simulink model "sampleModel7424_pp_1_1"  (R2018a)
settings: Solver=VariableStepAuto  StartTime=0.0  StopTime=10.0  RelTol=1e-3
undefined symbols (not defined in the file): DiscIntNeverNeededParam
libraries: simulink x211
(part 5 of 7)

== system sampleModel7424_pp_1_1/cfblk134/cfblk19 ==
  cfblk1 : Inport
  cfblk11 : Inport  Port=2
  cfblk12 : Inport  Port=3
  Action Port : ActionPort  ActionType=else
  cfblk10 : simulink/Continuous/PID Controller  Controller=PID  TimeDomain=Discrete-time  SampleTime=-1  IntegratorMethod=Forward Euler  FilterMethod=Forward Euler  Form=Parallel  UseFilter=on  ControllerParametersSource=internal  P=1  I=1  D=0  N=100  InitialConditionSource=internal  InitialConditionForIntegrator=0  InitialConditionForFilter=0  ExternalReset=none  LimitOutput=off  UpperSaturationLimit=inf  LowerSaturationLimit=-inf  LinearizeAsGain=off  AntiWindupMode=none  Kb=1  TrackingMode=off  Kt=1  PParamMin=[]  PParamMax=[]  IParamMin=[]  IParamMax=[]  DParamMin=[]  DParamMax=[]  NParamMin=[]  NParamMax=[]  KbParamMin=[]  KbParamMax=[]  KtParamMin=[]  KtParamMax=[]  POutMin=[]  POutMax=[]  IOutMin=[]  IOutMax=[]  DOutMin=[]  DOutMax=[]  NOutMin=[]  NOutMax=[]  KbOutMin=[]  KbOutMax=[]  KtOutMin=[]  KtOutMax=[]  IntegratorOutMin=[]  IntegratorOutMax=[]  FilterOutMin=[]  FilterOutMax=[]  SumOutMin=[]  SumOutMax=[]  SumI1OutMin=[]  SumI1OutMax=[]  SumI2OutMin=[]  SumI2OutMax=[]  SumI3OutMin=[]  SumI3OutMax=[]  SumDOutMin=[]  SumDOutMax=[]  SaturationOutMin=[]  SaturationOutMax=[]  IntegratorContinuousStateAttributes=''  IntegratorStateMustResolveToSignalObject=off  IntegratorRTWStateStorageClass=Auto  FilterContinuousStateAttributes=''  FilterStateMustResolveToSignalObject=off  FilterRTWStateStorageClass=Auto  DifferentiatorICPrevScaledInput=0  DifferentiatorOutMin=[]  DifferentiatorOutMax=[]  FilterDiffOutCoefMin=[]  FilterDiffOutCoefMax=[]  SumDenOutMin=[]  SumDenOutMax=[]  SumNumOutMin=[]  SumNumOutMax=[]  ReciprocalOutMin=[]  ReciprocalOutMax=[]  DivideOutMin=[]  DivideOutMax=[]  TunerSelectOption=Transfer Function Based (PID Tuner App)
  cfblk15 : Delay
  cfblk3 : simulink/Continuous/PID Controller (2DOF)  Controller=PID  TimeDomain=Discrete-time  SampleTime=-1  IntegratorMethod=Forward Euler  FilterMethod=Forward Euler  Form=Parallel  UseFilter=on  ControllerParametersSource=internal  P=1  I=1  D=0  N=100  b=1  c=1  InitialConditionSource=internal  InitialConditionForIntegrator=0  InitialConditionForFilter=0  ExternalReset=none  LimitOutput=off  UpperSaturationLimit=inf  LowerSaturationLimit=-inf  LinearizeAsGain=off  AntiWindupMode=none  Kb=1  TrackingMode=off  Kt=1  PParamMin=[]  PParamMax=[]  IParamMin=[]  IParamMax=[]  DParamMin=[]  DParamMax=[]  NParamMin=[]  NParamMax=[]  bParamMin=[]  bParamMax=[]  cParamMin=[]  cParamMax=[]  KbParamMin=[]  KbParamMax=[]  KtParamMin=[]  KtParamMax=[]  POutMin=[]  POutMax=[]  IOutMin=[]  IOutMax=[]  DOutMin=[]  DOutMax=[]  NOutMin=[]  NOutMax=[]  bOutMin=[]  bOutMax=[]  cOutMin=[]  cOutMax=[]  KbOutMin=[]  KbOutMax=[]  KtOutMin=[]  KtOutMax=[]  IntegratorOutMin=[]  IntegratorOutMax=[]  FilterOutMin=[]  FilterOutMax=[]  SumOutMin=[]  SumOutMax=[]  Sum1OutMin=[]  Sum1OutMax=[]  Sum2OutMin=[]  Sum2OutMax=[]  Sum3OutMin=[]  Sum3OutMax=[]  SumI1OutMin=[]  SumI1OutMax=[]  SumI2OutMin=[]  SumI2OutMax=[]  SumI3OutMin=[]  SumI3OutMax=[]  SumDOutMin=[]  SumDOutMax=[]  SaturationOutMin=[]  SaturationOutMax=[]  IntegratorContinuousStateAttributes=''  IntegratorStateMustResolveToSignalObject=off  IntegratorRTWStateStorageClass=Auto  FilterContinuousStateAttributes=''  FilterStateMustResolveToSignalObject=off  FilterRTWStateStorageClass=Auto  DifferentiatorICPrevScaledInput=0  DifferentiatorOutMin=[]  DifferentiatorOutMax=[]  FilterDiffOutCoefMin=[]  FilterDiffOutCoefMax=[]  SumDenOutMin=[]  SumDenOutMax=[]  SumNumOutMin=[]  SumNumOutMax=[]  ReciprocalOutMin=[]  ReciprocalOutMax=[]  DivideOutMin=[]  DivideOutMax=[]  TunerSelectOption=Transfer Function Based (PID Tuner App)
  cfblk4 : simulink/Continuous/PID Controller  Controller=PID  TimeDomain=Discrete-time  SampleTime=-1  IntegratorMethod=Forward Euler  FilterMethod=Forward Euler  Form=Parallel  UseFilter=on  ControllerParametersSource=internal  P=1  I=1  D=0  N=100  InitialConditionSource=internal  InitialConditionForIntegrator=0  InitialConditionForFilter=0  ExternalReset=none  LimitOutput=off  UpperSaturationLimit=inf  LowerSaturationLimit=-inf  LinearizeAsGain=off  AntiWindupMode=none  Kb=1  TrackingMode=off  Kt=1  PParamMin=[]  PParamMax=[]  IParamMin=[]  IParamMax=[]  DParamMin=[]  DParamMax=[]  NParamMin=[]  NParamMax=[]  KbParamMin=[]  KbParamMax=[]  KtParamMin=[]  KtParamMax=[]  POutMin=[]  POutMax=[]  IOutMin=[]  IOutMax=[]  DOutMin=[]  DOutMax=[]  NOutMin=[]  NOutMax=[]  KbOutMin=[]  KbOutMax=[]  KtOutMin=[]  KtOutMax=[]  IntegratorOutMin=[]  IntegratorOutMax=[]  FilterOutMin=[]  FilterOutMax=[]  SumOutMin=[]  SumOutMax=[]  SumI1OutMin=[]  SumI1OutMax=[]  SumI2OutMin=[]  SumI2OutMax=[]  SumI3OutMin=[]  SumI3OutMax=[]  SumDOutMin=[]  SumDOutMax=[]  SaturationOutMin=[]  SaturationOutMax=[]  IntegratorContinuousStateAttributes=''  IntegratorStateMustResolveToSignalObject=off  IntegratorRTWStateStorageClass=Auto  FilterContinuousStateAttributes=''  FilterStateMustResolveToSignalObject=off  FilterRTWStateStorageClass=Auto  DifferentiatorICPrevScaledInput=0  DifferentiatorOutMin=[]  DifferentiatorOutMax=[]  FilterDiffOutCoefMin=[]  FilterDiffOutCoefMax=[]  SumDenOutMin=[]  SumDenOutMax=[]  SumNumOutMin=[]  SumNumOutMax=[]  ReciprocalOutMin=[]  ReciprocalOutMax=[]  DivideOutMin=[]  DivideOutMax=[]  TunerSelectOption=Transfer Function Based (PID Tuner App)
  cfblk5 : DiscreteFir
  cfblk6 : DiscreteFilter
  cfblk7 : DiscreteFir
  cfblk8 : simulink/Discrete/Difference  ICPrevInput=0.0  OutMin=[]  OutMax=[]  OutDataTypeStr=double  OutputDataTypeScalingMode=double  OutDataType=fixdt(1, 16)  OutScaling=2^-10  DoSatur=off
  cfblk9 : simulink/Discrete/Tapped Delay  vinit=0.0  samptime=-1  NumDelays=1  DelayOrder=Oldest  includeCurrent=off
  cyemi_{417..426} (10 alike) : DataTypeConversion  OutDataTypeStr=double
  emi_{68,76,148,276,282,298} (6 alike) : UnaryMinus
  emi_149 : MATLAB Function  TreatAsAtomicUnit=on
  emi_277 : MATLAB Function  TreatAsAtomicUnit=on
  emi_283 : MATLAB Function  TreatAsAtomicUnit=on
  emi_299 : MATLAB Function  TreatAsAtomicUnit=on
  emi_69 : MATLAB Function  TreatAsAtomicUnit=on
  emi_77 : MATLAB Function  TreatAsAtomicUnit=on
  cfblk2 : Outport
  cfblk13 : Outport  Port=2
  cfblk14 : Outport  Port=3
  wires:
  cfblk4/1 -> cfblk13/1, cfblk2/1
  cfblk12/1 -> cfblk14/1
  cyemi_417/1 -> cfblk10/1, emi_276/1, emi_277/1(o)
  cfblk8/1 -> cyemi_417/1
  cyemi_418/1 -> cfblk15/1
  cfblk9/1 -> cyemi_418/1
  cyemi_419/1 -> cfblk3/1
  cfblk10/1 -> cyemi_419/1
  cyemi_420/1 -> cfblk3/2
  cfblk7/1 -> cyemi_420/1
  cyemi_421/1 -> cfblk4/1
  cfblk3/1 -> cyemi_421/1
  cyemi_422/1 -> cfblk5/1, emi_148/1, emi_149/1(o)
  cfblk15/1 -> cyemi_422/1
  cyemi_423/1 -> cfblk6/1, emi_282/1, emi_283/1(o)
  cfblk11/1 -> cyemi_423/1
  cyemi_424/1 -> cfblk7/1, emi_68/1, emi_69/1(o), emi_298/1, emi_299/1(o)
  cfblk1/1 -> cyemi_424/1
  cyemi_425/1 -> cfblk8/1
  cfblk6/1 -> cyemi_425/1
  cyemi_426/1 -> cfblk9/1, emi_76/1, emi_77/1(o)
  cfblk5/1 -> cyemi_426/1
  emi_68/1 -> emi_69/2(e)
  emi_76/1 -> emi_77/2(e)
  emi_148/1 -> emi_149/2(e)
  emi_276/1 -> emi_277/2(e)
  emi_282/1 -> emi_283/2(e)
  emi_298/1 -> emi_299/2(e)

== system sampleModel7424_pp_1_1/cfblk142/cfblk16 ==
  cfblk1 : Inport
  cfblk11 : Inport  Port=2
  Action Port : ActionPort  ActionType=then
  cfblk10 : simulink/Discrete/Transfer Fcn First Order  PoleZ=0.95  ICPrevOutput=0.0  DoSatur=off
      settings: SourceProductName=Simulink
  cfblk12 : Delay
  cfblk3 : simulink/Continuous/PID Controller (2DOF)  Controller=PID  TimeDomain=Discrete-time  SampleTime=-1  IntegratorMethod=Forward Euler  FilterMethod=Forward Euler  Form=Parallel  UseFilter=on  ControllerParametersSource=internal  P=1  I=1  D=0  N=100  b=1  c=1  InitialConditionSource=internal  InitialConditionForIntegrator=0  InitialConditionForFilter=0  ExternalReset=none  LimitOutput=off  UpperSaturationLimit=inf  LowerSaturationLimit=-inf  LinearizeAsGain=off  AntiWindupMode=none  Kb=1  TrackingMode=off  Kt=1  PParamMin=[]  PParamMax=[]  IParamMin=[]  IParamMax=[]  DParamMin=[]  DParamMax=[]  NParamMin=[]  NParamMax=[]  bParamMin=[]  bParamMax=[]  cParamMin=[]  cParamMax=[]  KbParamMin=[]  KbParamMax=[]  KtParamMin=[]  KtParamMax=[]  POutMin=[]  POutMax=[]  IOutMin=[]  IOutMax=[]  DOutMin=[]  DOutMax=[]  NOutMin=[]  NOutMax=[]  bOutMin=[]  bOutMax=[]  cOutMin=[]  cOutMax=[]  KbOutMin=[]  KbOutMax=[]  KtOutMin=[]  KtOutMax=[]  IntegratorOutMin=[]  IntegratorOutMax=[]  FilterOutMin=[]  FilterOutMax=[]  SumOutMin=[]  SumOutMax=[]  Sum1OutMin=[]  Sum1OutMax=[]  Sum2OutMin=[]  Sum2OutMax=[]  Sum3OutMin=[]  Sum3OutMax=[]  SumI1OutMin=[]  SumI1OutMax=[]  SumI2OutMin=[]  SumI2OutMax=[]  SumI3OutMin=[]  SumI3OutMax=[]  SumDOutMin=[]  SumDOutMax=[]  SaturationOutMin=[]  SaturationOutMax=[]  IntegratorContinuousStateAttributes=''  IntegratorStateMustResolveToSignalObject=off  IntegratorRTWStateStorageClass=Auto  FilterContinuousStateAttributes=''  FilterStateMustResolveToSignalObject=off  FilterRTWStateStorageClass=Auto  DifferentiatorICPrevScaledInput=0  DifferentiatorOutMin=[]  DifferentiatorOutMax=[]  FilterDiffOutCoefMin=[]  FilterDiffOutCoefMax=[]  SumDenOutMin=[]  SumDenOutMax=[]  SumNumOutMin=[]  SumNumOutMax=[]  ReciprocalOutMin=[]  ReciprocalOutMax=[]  DivideOutMin=[]  DivideOutMax=[]  TunerSelectOption=Transfer Function Based (PID Tuner App)
  cfblk4 : simulink/Continuous/PID Controller (2DOF)  Controller=PID  TimeDomain=Discrete-time  SampleTime=-1  IntegratorMethod=Forward Euler  FilterMethod=Forward Euler  Form=Parallel  UseFilter=on  ControllerParametersSource=internal  P=1  I=1  D=0  N=100  b=1  c=1  InitialConditionSource=internal  InitialConditionForIntegrator=0  InitialConditionForFilter=0  ExternalReset=none  LimitOutput=off  UpperSaturationLimit=inf  LowerSaturationLimit=-inf  LinearizeAsGain=off  AntiWindupMode=none  Kb=1  TrackingMode=off  Kt=1  PParamMin=[]  PParamMax=[]  IParamMin=[]  IParamMax=[]  DParamMin=[]  DParamMax=[]  NParamMin=[]  NParamMax=[]  bParamMin=[]  bParamMax=[]  cParamMin=[]  cParamMax=[]  KbParamMin=[]  KbParamMax=[]  KtParamMin=[]  KtParamMax=[]  POutMin=[]  POutMax=[]  IOutMin=[]  IOutMax=[]  DOutMin=[]  DOutMax=[]  NOutMin=[]  NOutMax=[]  bOutMin=[]  bOutMax=[]  cOutMin=[]  cOutMax=[]  KbOutMin=[]  KbOutMax=[]  KtOutMin=[]  KtOutMax=[]  IntegratorOutMin=[]  IntegratorOutMax=[]  FilterOutMin=[]  FilterOutMax=[]  SumOutMin=[]  SumOutMax=[]  Sum1OutMin=[]  Sum1OutMax=[]  Sum2OutMin=[]  Sum2OutMax=[]  Sum3OutMin=[]  Sum3OutMax=[]  SumI1OutMin=[]  SumI1OutMax=[]  SumI2OutMin=[]  SumI2OutMax=[]  SumI3OutMin=[]  SumI3OutMax=[]  SumDOutMin=[]  SumDOutMax=[]  SaturationOutMin=[]  SaturationOutMax=[]  IntegratorContinuousStateAttributes=''  IntegratorStateMustResolveToSignalObject=off  IntegratorRTWStateStorageClass=Auto  FilterContinuousStateAttributes=''  FilterStateMustResolveToSignalObject=off  FilterRTWStateStorageClass=Auto  DifferentiatorICPrevScaledInput=0  DifferentiatorOutMin=[]  DifferentiatorOutMax=[]  FilterDiffOutCoefMin=[]  FilterDiffOutCoefMax=[]  SumDenOutMin=[]  SumDenOutMax=[]  SumNumOutMin=[]  SumNumOutMax=[]  ReciprocalOutMin=[]  ReciprocalOutMax=[]  DivideOutMin=[]  DivideOutMax=[]  TunerSelectOption=Transfer Function Based (PID Tuner App)
  cfblk5 : Delay  DelayLengthSource=Input port
      settings: InputPortMap=u0,p1
  cfblk6 : simulink/Discrete/Tapped Delay  vinit=0.0  samptime=-1  NumDelays=1  DelayOrder=Oldest  includeCurrent=off
  cfblk7 : DiscreteFir
  cfblk8 : simulink/Discrete/Tapped Delay  vinit=0.0  samptime=-1  NumDelays=1  DelayOrder=Oldest  includeCurrent=off
  cfblk9 : simulink/Continuous/PID Controller (2DOF)  Controller=PID  TimeDomain=Discrete-time  SampleTime=-1  IntegratorMethod=Forward Euler  FilterMethod=Forward Euler  Form=Parallel  UseFilter=on  ControllerParametersSource=internal  P=1  I=1  D=0  N=100  b=1  c=1  InitialConditionSource=internal  InitialConditionForIntegrator=0  InitialConditionForFilter=0  ExternalReset=none  LimitOutput=off  UpperSaturationLimit=inf  LowerSaturationLimit=-inf  LinearizeAsGain=off  AntiWindupMode=none  Kb=1  TrackingMode=off  Kt=1  PParamMin=[]  PParamMax=[]  IParamMin=[]  IParamMax=[]  DParamMin=[]  DParamMax=[]  NParamMin=[]  NParamMax=[]  bParamMin=[]  bParamMax=[]  cParamMin=[]  cParamMax=[]  KbParamMin=[]  KbParamMax=[]  KtParamMin=[]  KtParamMax=[]  POutMin=[]  POutMax=[]  IOutMin=[]  IOutMax=[]  DOutMin=[]  DOutMax=[]  NOutMin=[]  NOutMax=[]  bOutMin=[]  bOutMax=[]  cOutMin=[]  cOutMax=[]  KbOutMin=[]  KbOutMax=[]  KtOutMin=[]  KtOutMax=[]  IntegratorOutMin=[]  IntegratorOutMax=[]  FilterOutMin=[]  FilterOutMax=[]  SumOutMin=[]  SumOutMax=[]  Sum1OutMin=[]  Sum1OutMax=[]  Sum2OutMin=[]  Sum2OutMax=[]  Sum3OutMin=[]  Sum3OutMax=[]  SumI1OutMin=[]  SumI1OutMax=[]  SumI2OutMin=[]  SumI2OutMax=[]  SumI3OutMin=[]  SumI3OutMax=[]  SumDOutMin=[]  SumDOutMax=[]  SaturationOutMin=[]  SaturationOutMax=[]  IntegratorContinuousStateAttributes=''  IntegratorStateMustResolveToSignalObject=off  IntegratorRTWStateStorageClass=Auto  FilterContinuousStateAttributes=''  FilterStateMustResolveToSignalObject=off  FilterRTWStateStorageClass=Auto  DifferentiatorICPrevScaledInput=0  DifferentiatorOutMin=[]  DifferentiatorOutMax=[]  FilterDiffOutCoefMin=[]  FilterDiffOutCoefMax=[]  SumDenOutMin=[]  SumDenOutMax=[]  SumNumOutMin=[]  SumNumOutMax=[]  ReciprocalOutMin=[]  ReciprocalOutMax=[]  DivideOutMin=[]  DivideOutMax=[]  TunerSelectOption=Transfer Function Based (PID Tuner App)
  cyemi_{528..540} (13 alike) : DataTypeConversion  OutDataTypeStr=double
  cfblk2 : Outport
  wires:
  cfblk9/1 -> cyemi_532/1, cyemi_538/1
  cfblk7/1 -> cyemi_528/1, cyemi_529/1
  cfblk5/1 -> cfblk2/1
  cfblk11/1 -> cyemi_533/1, cyemi_540/1
  cyemi_528/1 -> cfblk10/1
  cyemi_529/1 -> cfblk12/1
  cyemi_530/1 -> cfblk3/1
  cfblk1/1 -> cyemi_530/1
  cyemi_531/1 -> cfblk3/2
  cfblk12/1 -> cyemi_531/1
  cyemi_532/1 -> cfblk4/1
  cyemi_533/1 -> cfblk4/2
  cyemi_534/1 -> cfblk5/1
  cfblk8/1 -> cyemi_534/1
  cyemi_535/1 -> cfblk5/2
  cfblk4/1 -> cyemi_535/1
  cyemi_536/1 -> cfblk6/1
  cfblk3/1 -> cyemi_536/1
  cyemi_537/1 -> cfblk7/1
  cfblk6/1 -> cyemi_537/1
  cyemi_538/1 -> cfblk8/1
  cyemi_539/1 -> cfblk9/1
  cfblk10/1 -> cyemi_539/1
  cyemi_540/1 -> cfblk9/2

== system sampleModel7424_pp_1_1/cfblk142/cfblk17 ==
  cfblk1 : Inport
  Action Port : ActionPort  ActionType=else
  cfblk3 : simulink/Discrete/Difference  ICPrevInput=0.0  OutMin=[]  OutMax=[]  OutDataTypeStr=double  OutputDataTypeScalingMode=double  OutDataType=fixdt(1, 16)  OutScaling=2^-10  DoSatur=off
  cfblk4 : simulink/Discrete/Transfer Fcn Real Zero  ZeroZ=0.75  ICPrevInput=0.0  DoSatur=off
      settings: SourceProductName=Simulink  SourceProductBaseCode=SL
  cfblk5 : simulink/Discrete/Tapped Delay  vinit=0.0  samptime=-1  NumDelays=1  DelayOrder=Oldest  includeCurrent=off
  cfblk6 : simulink/Discrete/Transfer Fcn First Order  PoleZ=0.95  ICPrevOutput=0.0  DoSatur=off
      settings: SourceProductName=Simulink
  cfblk8 : Delay
  cyemi_{542..546} (5 alike) : DataTypeConversion  OutDataTypeStr=double
  emi_0 : UnaryMinus
  emi_1 : MATLAB Function  TreatAsAtomicUnit=on
  emi_74 : UnaryMinus
  emi_75 : MATLAB Function  TreatAsAtomicUnit=on
  emi_80 : UnaryMinus
  emi_81 : MATLAB Function  TreatAsAtomicUnit=on
  cfblk2 : Outport
  cfblk7 : Outport  Port=2
  wires:
  cfblk5/1 -> cfblk2/1
  cfblk1/1 -> cfblk7/1
  cfblk4/1 -> cyemi_544/1, cyemi_545/1
  cyemi_542/1 -> cfblk3/1, emi_80/1, emi_81/1(o)
  cfblk8/1 -> cyemi_542/1
  cyemi_543/1 -> cfblk4/1, emi_0/1, emi_1/1(o)
  cfblk3/1 -> cyemi_543/1
  cyemi_544/1 -> cfblk5/1
  cyemi_545/1 -> cfblk6/1
  cyemi_546/1 -> cfblk8/1, emi_74/1, emi_75/1(o)
  cfblk6/1 -> cyemi_546/1
  emi_0/1 -> emi_1/2(e)
  emi_74/1 -> emi_75/2(e)
  emi_80/1 -> emi_81/2(e)

== system sampleModel7424_pp_1_1/cfblk142/cfblk18 ==
  cfblk1 : Inport
  Action Port : ActionPort  ActionType=then
  cfblk10 : Delay  DelayLengthSource=Input port
      settings: InputPortMap=u0,p1
  cfblk11 : DiscreteStateSpace  SampleTime=-1
  cfblk12 : DiscreteFilter
  cfblk13 : simulink/Continuous/PID Controller  Controller=PID  TimeDomain=Discrete-time  SampleTime=-1  IntegratorMethod=Forward Euler  FilterMethod=Forward Euler  Form=Parallel  UseFilter=on  ControllerParametersSource=internal  P=1  I=1  D=0  N=100  InitialConditionSource=internal  InitialConditionForIntegrator=0  InitialConditionForFilter=0  ExternalReset=none  LimitOutput=off  UpperSaturationLimit=inf  LowerSaturationLimit=-inf  LinearizeAsGain=off  AntiWindupMode=none  Kb=1  TrackingMode=off  Kt=1  PParamMin=[]  PParamMax=[]  IParamMin=[]  IParamMax=[]  DParamMin=[]  DParamMax=[]  NParamMin=[]  NParamMax=[]  KbParamMin=[]  KbParamMax=[]  KtParamMin=[]  KtParamMax=[]  POutMin=[]  POutMax=[]  IOutMin=[]  IOutMax=[]  DOutMin=[]  DOutMax=[]  NOutMin=[]  NOutMax=[]  KbOutMin=[]  KbOutMax=[]  KtOutMin=[]  KtOutMax=[]  IntegratorOutMin=[]  IntegratorOutMax=[]  FilterOutMin=[]  FilterOutMax=[]  SumOutMin=[]  SumOutMax=[]  SumI1OutMin=[]  SumI1OutMax=[]  SumI2OutMin=[]  SumI2OutMax=[]  SumI3OutMin=[]  SumI3OutMax=[]  SumDOutMin=[]  SumDOutMax=[]  SaturationOutMin=[]  SaturationOutMax=[]  IntegratorContinuousStateAttributes=''  IntegratorStateMustResolveToSignalObject=off  IntegratorRTWStateStorageClass=Auto  FilterContinuousStateAttributes=''  FilterStateMustResolveToSignalObject=off  FilterRTWStateStorageClass=Auto  DifferentiatorICPrevScaledInput=0  DifferentiatorOutMin=[]  DifferentiatorOutMax=[]  FilterDiffOutCoefMin=[]  FilterDiffOutCoefMax=[]  SumDenOutMin=[]  SumDenOutMax=[]  SumNumOutMin=[]  SumNumOutMax=[]  ReciprocalOutMin=[]  ReciprocalOutMax=[]  DivideOutMin=[]  DivideOutMax=[]  TunerSelectOption=Transfer Function Based (PID Tuner App)
  cfblk{5,16..18} (4 alike) : Delay
  cfblk3 : Delay  ShowEnablePort=on
      settings: InputPortMap=u0,e6
  cfblk4 : simulink/Continuous/PID Controller (2DOF)  Controller=PID  TimeDomain=Discrete-time  SampleTime=-1  IntegratorMethod=Forward Euler  FilterMethod=Forward Euler  Form=Parallel  UseFilter=on  ControllerParametersSource=internal  P=1  I=1  D=0  N=100  b=1  c=1  InitialConditionSource=internal  InitialConditionForIntegrator=0  InitialConditionForFilter=0  ExternalReset=none  LimitOutput=off  UpperSaturationLimit=inf  LowerSaturationLimit=-inf  LinearizeAsGain=off  AntiWindupMode=none  Kb=1  TrackingMode=off  Kt=1  PParamMin=[]  PParamMax=[]  IParamMin=[]  IParamMax=[]  DParamMin=[]  DParamMax=[]  NParamMin=[]  NParamMax=[]  bParamMin=[]  bParamMax=[]  cParamMin=[]  cParamMax=[]  KbParamMin=[]  KbParamMax=[]  KtParamMin=[]  KtParamMax=[]  POutMin=[]  POutMax=[]  IOutMin=[]  IOutMax=[]  DOutMin=[]  DOutMax=[]  NOutMin=[]  NOutMax=[]  bOutMin=[]  bOutMax=[]  cOutMin=[]  cOutMax=[]  KbOutMin=[]  KbOutMax=[]  KtOutMin=[]  KtOutMax=[]  IntegratorOutMin=[]  IntegratorOutMax=[]  FilterOutMin=[]  FilterOutMax=[]  SumOutMin=[]  SumOutMax=[]  Sum1OutMin=[]  Sum1OutMax=[]  Sum2OutMin=[]  Sum2OutMax=[]  Sum3OutMin=[]  Sum3OutMax=[]  SumI1OutMin=[]  SumI1OutMax=[]  SumI2OutMin=[]  SumI2OutMax=[]  SumI3OutMin=[]  SumI3OutMax=[]  SumDOutMin=[]  SumDOutMax=[]  SaturationOutMin=[]  SaturationOutMax=[]  IntegratorContinuousStateAttributes=''  IntegratorStateMustResolveToSignalObject=off  IntegratorRTWStateStorageClass=Auto  FilterContinuousStateAttributes=''  FilterStateMustResolveToSignalObject=off  FilterRTWStateStorageClass=Auto  DifferentiatorICPrevScaledInput=0  DifferentiatorOutMin=[]  DifferentiatorOutMax=[]  FilterDiffOutCoefMin=[]  FilterDiffOutCoefMax=[]  SumDenOutMin=[]  SumDenOutMax=[]  SumNumOutMin=[]  SumNumOutMax=[]  ReciprocalOutMin=[]  ReciprocalOutMax=[]  DivideOutMin=[]  DivideOutMax=[]  TunerSelectOption=Transfer Function Based (PID Tuner App)
  cfblk6 : DiscreteTransferFcn
  cfblk7 : DiscreteTransferFcn
  cfblk8 : DiscreteFilter
  cfblk9 : DiscreteFir
  cyemi_{548..564} (17 alike) : DataTypeConversion  OutDataTypeStr=double
  cfblk2 : Outport
  cfblk14 : Outport  Port=2
  cfblk15 : Outport  Port=3
  wires:
  cfblk6/1 -> cfblk2/1
  cfblk5/1 -> cfblk14/1
  cfblk4/1 -> cfblk15/1
  cfblk9/1 -> cyemi_554/1, cyemi_555/1, cyemi_562/1
  cfblk11/1 -> cyemi_551/1, cyemi_558/1, cyemi_561/1
  cfblk7/1 -> cyemi_552/1, cyemi_553/1
  cyemi_548/1 -> cfblk10/1
  cfblk12/1 -> cyemi_548/1
  cyemi_549/1 -> cfblk10/2
  cfblk17/1 -> cyemi_549/1
  cyemi_550/1 -> cfblk11/1
  cfblk3/1 -> cyemi_550/1
  cyemi_551/1 -> cfblk12/1
  cyemi_552/1 -> cfblk13/1
  cyemi_553/1 -> cfblk16/1
  cyemi_554/1 -> cfblk17/1
  cyemi_555/1 -> cfblk18/1
  cyemi_556/1 -> cfblk3/1
  cfblk16/1 -> cyemi_556/1
  cyemi_557/1 -> cfblk3/2
  cfblk18/1 -> cyemi_557/1
  cyemi_558/1 -> cfblk4/1
  cyemi_559/1 -> cfblk4/2
  cfblk8/1 -> cyemi_559/1
  cyemi_560/1 -> cfblk5/1
  cfblk1/1 -> cyemi_560/1
  cyemi_561/1 -> cfblk6/1
  cyemi_562/1 -> cfblk7/1
  cyemi_563/1 -> cfblk8/1
  cfblk13/1 -> cyemi_563/1
  cyemi_564/1 -> cfblk9/1
  cfblk10/1 -> cyemi_564/1

== system sampleModel7424_pp_1_1/cfblk142/cfblk19 ==
  cfblk1 : Inport
  cfblk11 : Inport  Port=2
  Action Port : ActionPort  ActionType=else
  cfblk10 : DiscreteStateSpace  SampleTime=-1
  cfblk14 : Delay
  cfblk3 : simulink/Discrete/Transfer Fcn Real Zero  ZeroZ=0.75  ICPrevInput=0.0  DoSatur=off
      settings: SourceProductName=Simulink  SourceProductBaseCode=SL
  cfblk4 : DiscreteFilter
  cfblk5 : Delay  DelayLengthSource=Input port
      settings: InputPortMap=u0,p1
  cfblk6 : simulink/Continuous/PID Controller  Controller=PID  TimeDomain=Discrete-time  SampleTime=-1  IntegratorMethod=Forward Euler  FilterMethod=Forward Euler  Form=Parallel  UseFilter=on  ControllerParametersSource=internal  P=1  I=1  D=0  N=100  InitialConditionSource=internal  InitialConditionForIntegrator=0  InitialConditionForFilter=0  ExternalReset=none  LimitOutput=off  UpperSaturationLimit=inf  LowerSaturationLimit=-inf  LinearizeAsGain=off  AntiWindupMode=none  Kb=1  TrackingMode=off  Kt=1  PParamMin=[]  PParamMax=[]  IParamMin=[]  IParamMax=[]  DParamMin=[]  DParamMax=[]  NParamMin=[]  NParamMax=[]  KbParamMin=[]  KbParamMax=[]  KtParamMin=[]  KtParamMax=[]  POutMin=[]  POutMax=[]  IOutMin=[]  IOutMax=[]  DOutMin=[]  DOutMax=[]  NOutMin=[]  NOutMax=[]  KbOutMin=[]  KbOutMax=[]  KtOutMin=[]  KtOutMax=[]  IntegratorOutMin=[]  IntegratorOutMax=[]  FilterOutMin=[]  FilterOutMax=[]  SumOutMin=[]  SumOutMax=[]  SumI1OutMin=[]  SumI1OutMax=[]  SumI2OutMin=[]  SumI2OutMax=[]  SumI3OutMin=[]  SumI3OutMax=[]  SumDOutMin=[]  SumDOutMax=[]  SaturationOutMin=[]  SaturationOutMax=[]  IntegratorContinuousStateAttributes=''  IntegratorStateMustResolveToSignalObject=off  IntegratorRTWStateStorageClass=Auto  FilterContinuousStateAttributes=''  FilterStateMustResolveToSignalObject=off  FilterRTWStateStorageClass=Auto  DifferentiatorICPrevScaledInput=0  DifferentiatorOutMin=[]  DifferentiatorOutMax=[]  FilterDiffOutCoefMin=[]  FilterDiffOutCoefMax=[]  SumDenOutMin=[]  SumDenOutMax=[]  SumNumOutMin=[]  SumNumOutMax=[]  ReciprocalOutMin=[]  ReciprocalOutMax=[]  DivideOutMin=[]  DivideOutMax=[]  TunerSelectOption=Transfer Function Based (PID Tuner App)
  cfblk7 : DiscreteZeroPole  Poles=[0 0.5]  Gain=1  SampleTime=-1
  cfblk8 : DiscreteFilter
  cfblk9 : simulink/Discrete/Tapped Delay  vinit=0.0  samptime=-1  NumDelays=1  DelayOrder=Oldest  includeCurrent=off
  cyemi_{567..576} (10 alike) : DataTypeConversion  OutDataTypeStr=double
  emi_{8,10,56,86,170,212} (6 alike) : UnaryMinus
  emi_11 : MATLAB Function  TreatAsAtomicUnit=on
  emi_171 : MATLAB Function  TreatAsAtomicUnit=on
  emi_213 : MATLAB Function  TreatAsAtomicUnit=on
  emi_57 : MATLAB Function  TreatAsAtomicUnit=on
  emi_87 : MATLAB Function  TreatAsAtomicUnit=on
  emi_9 : MATLAB Function  TreatAsAtomicUnit=on
  cfblk2 : Outport
  cfblk12 : Outport  Port=2
  cfblk13 : Outport  Port=3
  wires:
  cfblk4/1 -> cfblk2/1, cfblk13/1
  cfblk8/1 -> cfblk12/1, cyemi_572/1
  cyemi_567/1 -> cfblk10/1
  cfblk3/1 -> cyemi_567/1
  cyemi_568/1 -> cfblk14/1
  cfblk7/1 -> cyemi_568/1
  cyemi_569/1 -> cfblk3/1, emi_8/1, emi_9/1(o), emi_86/1, emi_87/1(o)
  cfblk9/1 -> cyemi_569/1
  cyemi_570/1 -> cfblk4/1
  cfblk11/1 -> cyemi_570/1
  cyemi_571/1 -> cfblk5/1, emi_10/1, emi_11/1(o), emi_170/1, emi_171/1(o), emi_212/1, emi_213/1(o)
  cfblk14/1 -> cyemi_571/1
  cyemi_572/1 -> cfblk5/2
  cyemi_573/1 -> cfblk6/1
  cfblk10/1 -> cyemi_573/1
  cyemi_574/1 -> cfblk7/1
  cfblk6/1 -> cyemi_574/1
  cyemi_575/1 -> cfblk8/1
  cfblk1/1 -> cyemi_575/1
  cyemi_576/1 -> cfblk9/1, emi_56/1, emi_57/1(o)
  cfblk5/1 -> cyemi_576/1
  emi_8/1 -> emi_9/2(e)
  emi_10/1 -> emi_11/2(e)
  emi_56/1 -> emi_57/2(e)
  emi_86/1 -> emi_87/2(e)
  emi_170/1 -> emi_171/2(e)
  emi_212/1 -> emi_213/2(e)

== system sampleModel7424_pp_1_1/cfblk145/cfblk17 ==
  cfblk1 : Inport
  cfblk14 : Inport  Port=2
  cfblk15 : Inport  Port=3
  cfblk16 : Inport  Port=4
  Action Port : ActionPort  ActionType=then
  cfblk10 : DiscreteTransferFcn
  cfblk{3,5,11,13} (4 alike) : Delay  DelayLengthSource=Input port
      settings: InputPortMap=u0,p1
  cfblk12 : simulink/Discrete/Transfer Fcn Lead or Lag  PoleZ=0.95  ZeroZ=0.75  ICPrevOutput=0.0  ICPrevInput=0.0  DoSatur=off
      settings: SourceProductName=Simulink  SourceProductBaseCode=SL
  cfblk18 : Delay
  cfblk19 : DataTypeConversion  OutDataTypeStr=double
  cfblk20 : DataTypeConversion  OutDataTypeStr=double
  cfblk21 : DataTypeConversion  OutDataTypeStr=uint32
  cfblk22 : DataTypeConversion  OutDataTypeStr=double
  cfblk4 : DiscreteIntegrator  SampleTime=-1  OutDataTypeStr=double  ICPrevOutput=DiscIntNeverNeededParam  ICPrevScaledInput=DiscIntNeverNeededParam
  cfblk6 : DiscreteTransferFcn
  cfblk7 : simulink/Continuous/PID Controller (2DOF)  Controller=PID  TimeDomain=Discrete-time  SampleTime=-1  IntegratorMethod=Forward Euler  FilterMethod=Forward Euler  Form=Parallel  UseFilter=on  ControllerParametersSource=internal  P=1  I=1  D=0  N=100  b=1  c=1  InitialConditionSource=internal  InitialConditionForIntegrator=0  InitialConditionForFilter=0  ExternalReset=none  LimitOutput=off  UpperSaturationLimit=inf  LowerSaturationLimit=-inf  LinearizeAsGain=off  AntiWindupMode=none  Kb=1  TrackingMode=off  Kt=1  PParamMin=[]  PParamMax=[]  IParamMin=[]  IParamMax=[]  DParamMin=[]  DParamMax=[]  NParamMin=[]  NParamMax=[]  bParamMin=[]  bParamMax=[]  cParamMin=[]  cParamMax=[]  KbParamMin=[]  KbParamMax=[]  KtParamMin=[]  KtParamMax=[]  POutMin=[]  POutMax=[]  IOutMin=[]  IOutMax=[]  DOutMin=[]  DOutMax=[]  NOutMin=[]  NOutMax=[]  bOutMin=[]  bOutMax=[]  cOutMin=[]  cOutMax=[]  KbOutMin=[]  KbOutMax=[]  KtOutMin=[]  KtOutMax=[]  IntegratorOutMin=[]  IntegratorOutMax=[]  FilterOutMin=[]  FilterOutMax=[]  SumOutMin=[]  SumOutMax=[]  Sum1OutMin=[]  Sum1OutMax=[]  Sum2OutMin=[]  Sum2OutMax=[]  Sum3OutMin=[]  Sum3OutMax=[]  SumI1OutMin=[]  SumI1OutMax=[]  SumI2OutMin=[]  SumI2OutMax=[]  SumI3OutMin=[]  SumI3OutMax=[]  SumDOutMin=[]  SumDOutMax=[]  SaturationOutMin=[]  SaturationOutMax=[]  IntegratorContinuousStateAttributes=''  IntegratorStateMustResolveToSignalObject=off  IntegratorRTWStateStorageClass=Auto  FilterContinuousStateAttributes=''  FilterStateMustResolveToSignalObject=off  FilterRTWStateStorageClass=Auto  DifferentiatorICPrevScaledInput=0  DifferentiatorOutMin=[]  DifferentiatorOutMax=[]  FilterDiffOutCoefMin=[]  FilterDiffOutCoefMax=[]  SumDenOutMin=[]  SumDenOutMax=[]  SumNumOutMin=[]  SumNumOutMax=[]  ReciprocalOutMin=[]  ReciprocalOutMax=[]  DivideOutMin=[]  DivideOutMax=[]  TunerSelectOption=Transfer Function Based (PID Tuner App)
  cfblk8 : DiscreteFir
  cfblk9 : simulink/Discrete/Transfer Fcn Real Zero  ZeroZ=0.75  ICPrevInput=0.0  DoSatur=off
      settings: SourceProductName=Simulink  SourceProductBaseCode=SL
  cyemi_{626..627,629..633,635..646} (19 alike) : DataTypeConversion  OutDataTypeStr=double
  cyemi_628 : DataTypeConversion  OutDataTypeStr=uint32
  cyemi_634 : DataTypeConversion  OutDataTypeStr=uint32
  cfblk2 : Outport
  cfblk17 : Outport  Port=2
  wires:
  cfblk3/1 -> cfblk2/1
  cfblk1/1 -> cyemi_638/1, cyemi_641/1
  cfblk11/1 -> cfblk17/1
  cfblk8/1 -> cyemi_632/1, cyemi_636/1
  cfblk21/1 -> cyemi_628/1, cyemi_634/1
  cyemi_626/1 -> cfblk10/1
  cfblk16/1 -> cyemi_626/1
  cyemi_627/1 -> cfblk11/1
  cfblk10/1 -> cyemi_627/1
  cyemi_628/1 -> cfblk11/2
  cyemi_629/1 -> cfblk12/1
  cfblk22/1 -> cyemi_629/1
  cyemi_630/1 -> cfblk13/1
  cfblk19/1 -> cyemi_630/1
  cyemi_631/1 -> cfblk13/2
  cfblk4/1 -> cyemi_631/1
  cyemi_632/1 -> cfblk18/1
  cyemi_633/1 -> cfblk19/1
  cfblk9/1 -> cyemi_633/1
  cyemi_634/1 -> cfblk20/1
  cyemi_635/1 -> cfblk21/1
  cfblk12/1 -> cyemi_635/1
  cyemi_636/1 -> cfblk22/1
  cyemi_637/1 -> cfblk3/1
  cfblk13/1 -> cyemi_637/1
  cyemi_638/1 -> cfblk3/2
  cyemi_639/1 -> cfblk4/1
  cfblk7/1 -> cyemi_639/1
  cyemi_640/1 -> cfblk5/1
  cfblk14/1 -> cyemi_640/1
  cyemi_641/1 -> cfblk5/2
  cyemi_642/1 -> cfblk6/1
  cfblk18/1 -> cyemi_642/1
  cyemi_643/1 -> cfblk7/1
  cfblk15/1 -> cyemi_643/1
  cyemi_644/1 -> cfblk7/2
  cfblk5/1 -> cyemi_644/1
  cyemi_645/1 -> cfblk8/1
  cfblk6/1 -> cyemi_645/1
  cyemi_646/1 -> cfblk9/1
  cfblk20/1 -> cyemi_646/1

== system sampleModel7424_pp_1_1/cfblk145/cfblk18 ==
  cfblk1 : Inport
  cfblk15 : Inport  Port=2
  Action Port : ActionPort  ActionType=else
  cfblk10 : DiscreteStateSpace  SampleTime=-1
  cfblk11 : DiscreteIntegrator  SampleTime=-1  OutDataTypeStr=double  ICPrevOutput=DiscIntNeverNeededParam  ICPrevScaledInput=DiscIntNeverNeededParam
  cfblk12 : Delay  DelayLengthSource=Input port
      settings: InputPortMap=u0,p1
  cfblk13 : simulink/Continuous/PID Controller  Controller=PID  TimeDomain=Discrete-time  SampleTime=-1  IntegratorMethod=Forward Euler  FilterMethod=Forward Euler  Form=Parallel  UseFilter=on  ControllerParametersSource=internal  P=1  I=1  D=0  N=100  InitialConditionSource=internal  InitialConditionForIntegrator=0  InitialConditionForFilter=0  ExternalReset=none  LimitOutput=off  UpperSaturationLimit=inf  LowerSaturationLimit=-inf  LinearizeAsGain=off  AntiWindupMode=none  Kb=1  TrackingMode=off  Kt=1  PParamMin=[]  PParamMax=[]  IParamMin=[]  IParamMax=[]  DParamMin=[]  DParamMax=[]  NParamMin=[]  NParamMax=[]  KbParamMin=[]  KbParamMax=[]  KtParamMin=[]  KtParamMax=[]  POutMin=[]  POutMax=[]  IOutMin=[]  IOutMax=[]  DOutMin=[]  DOutMax=[]  NOutMin=[]  NOutMax=[]  KbOutMin=[]  KbOutMax=[]  KtOutMin=[]  KtOutMax=[]  IntegratorOutMin=[]  IntegratorOutMax=[]  FilterOutMin=[]  FilterOutMax=[]  SumOutMin=[]  SumOutMax=[]  SumI1OutMin=[]  SumI1OutMax=[]  SumI2OutMin=[]  SumI2OutMax=[]  SumI3OutMin=[]  SumI3OutMax=[]  SumDOutMin=[]  SumDOutMax=[]  SaturationOutMin=[]  SaturationOutMax=[]  IntegratorContinuousStateAttributes=''  IntegratorStateMustResolveToSignalObject=off  IntegratorRTWStateStorageClass=Auto  FilterContinuousStateAttributes=''  FilterStateMustResolveToSignalObject=off  FilterRTWStateStorageClass=Auto  DifferentiatorICPrevScaledInput=0  DifferentiatorOutMin=[]  DifferentiatorOutMax=[]  FilterDiffOutCoefMin=[]  FilterDiffOutCoefMax=[]  SumDenOutMin=[]  SumDenOutMax=[]  SumNumOutMin=[]  SumNumOutMax=[]  ReciprocalOutMin=[]  ReciprocalOutMax=[]  DivideOutMin=[]  DivideOutMax=[]  TunerSelectOption=Transfer Function Based (PID Tuner App)
  cfblk14 : simulink/Discrete/Difference  ICPrevInput=0.0  OutMin=[]  OutMax=[]  OutDataTypeStr=double  OutputDataTypeScalingMode=double  OutDataType=fixdt(1, 16)  OutScaling=2^-10  DoSatur=off
  cfblk16 : Delay
  cfblk17 : Delay
  cfblk18 : Delay
  cfblk3 : DiscreteFilter
  cfblk4 : Delay  ShowEnablePort=on
      settings: InputPortMap=u0,e6
  cfblk5 : DiscreteTransferFcn
  cfblk6 : simulink/Discrete/Transfer Fcn Lead or Lag  PoleZ=0.95  ZeroZ=0.75  ICPrevOutput=0.0  ICPrevInput=0.0  DoSatur=off
      settings: SourceProductName=Simulink  SourceProductBaseCode=SL
  cfblk7 : simulink/Discrete/Transfer Fcn Real Zero  ZeroZ=0.75  ICPrevInput=0.0  DoSatur=off
      settings: SourceProductName=Simulink  SourceProductBaseCode=SL
  cfblk8 : Delay  DelayLengthSource=Input port
      settings: InputPortMap=u0,p1
  cfblk9 : DiscreteIntegrator  SampleTime=-1  OutDataTypeStr=double  ICPrevOutput=DiscIntNeverNeededParam  ICPrevScaledInput=DiscIntNeverNeededParam
  cyemi_{649..666} (18 alike) : DataTypeConversion  OutDataTypeStr=double
  cfblk2 : Outport
  wires:
  cfblk11/1 -> cyemi_657/1, cyemi_664/1, cyemi_665/1
  cfblk3/1 -> cfblk2/1
  cyemi_649/1 -> cfblk10/1
  cfblk12/1 -> cyemi_649/1
  cyemi_650/1 -> cfblk11/1
  cfblk7/1 -> cyemi_650/1
  cyemi_651/1 -> cfblk12/1
  cfblk13/1 -> cyemi_651/1
  cyemi_652/1 -> cfblk12/2
  cfblk4/1 -> cyemi_652/1
  cyemi_653/1 -> cfblk13/1
  cfblk8/1 -> cyemi_653/1
  cyemi_654/1 -> cfblk14/1
  cfblk15/1 -> cyemi_654/1
  cyemi_655/1 -> cfblk16/1
  cfblk10/1 -> cyemi_655/1
  cyemi_656/1 -> cfblk17/1
  cfblk9/1 -> cyemi_656/1
  cyemi_657/1 -> cfblk18/1
  cyemi_658/1 -> cfblk3/1
  cfblk14/1 -> cyemi_658/1
  cyemi_659/1 -> cfblk4/1
  cfblk5/1 -> cyemi_659/1
  cyemi_660/1 -> cfblk4/2
  cfblk16/1 -> cyemi_660/1
  cyemi_661/1 -> cfblk5/1
  cfblk1/1 -> cyemi_661/1
  cyemi_662/1 -> cfblk6/1
  cfblk17/1 -> cyemi_662/1
  cyemi_663/1 -> cfblk7/1
  cfblk18/1 -> cyemi_663/1
  cyemi_664/1 -> cfblk8/1
  cyemi_665/1 -> cfblk8/2
  cyemi_666/1 -> cfblk9/1
  cfblk6/1 -> cyemi_666/1

== system sampleModel7424_pp_1_1/cfblk145/cfblk19 ==
  cfblk1 : Inport
  cfblk11 : Inport  Port=2
  Action Port : ActionPort  ActionType=then
  cfblk10 : DiscreteIntegrator  SampleTime=-1  OutDataTypeStr=double  ICPrevOutput=DiscIntNeverNeededParam  ICPrevScaledInput=DiscIntNeverNeededParam
  cfblk3 : UnitDelay  SampleTime=-1
  cfblk4 : simulink/Discrete/Difference  ICPrevInput=0.0  OutMin=[]  OutMax=[]  OutDataTypeStr=double  OutputDataTypeScalingMode=double  OutDataType=fixdt(1, 16)  OutScaling=2^-10  DoSatur=off
  cfblk5 : simulink/Discrete/Tapped Delay  vinit=0.0  samptime=-1  NumDelays=1  DelayOrder=Oldest  includeCurrent=off
  cfblk6 : simulink/Discrete/Transfer Fcn Real Zero  ZeroZ=0.75  ICPrevInput=0.0  DoSatur=off
      settings: SourceProductName=Simulink  SourceProductBaseCode=SL
  cfblk7 : simulink/Discrete/Tapped Delay  vinit=0.0  samptime=-1  NumDelays=1  DelayOrder=Oldest  includeCurrent=off
  cfblk8 : DiscreteStateSpace  SampleTime=-1
  cfblk9 : simulink/Continuous/PID Controller  Controller=PID  TimeDomain=Discrete-time  SampleTime=-1  IntegratorMethod=Forward Euler  FilterMethod=Forward Euler  Form=Parallel  UseFilter=on  ControllerParametersSource=internal  P=1  I=1  D=0  N=100  InitialConditionSource=internal  InitialConditionForIntegrator=0  InitialConditionForFilter=0  ExternalReset=none  LimitOutput=off  UpperSaturationLimit=inf  LowerSaturationLimit=-inf  LinearizeAsGain=off  AntiWindupMode=none  Kb=1  TrackingMode=off  Kt=1  PParamMin=[]  PParamMax=[]  IParamMin=[]  IParamMax=[]  DParamMin=[]  DParamMax=[]  NParamMin=[]  NParamMax=[]  KbParamMin=[]  KbParamMax=[]  KtParamMin=[]  KtParamMax=[]  POutMin=[]  POutMax=[]  IOutMin=[]  IOutMax=[]  DOutMin=[]  DOutMax=[]  NOutMin=[]  NOutMax=[]  KbOutMin=[]  KbOutMax=[]  KtOutMin=[]  KtOutMax=[]  IntegratorOutMin=[]  IntegratorOutMax=[]  FilterOutMin=[]  FilterOutMax=[]  SumOutMin=[]  SumOutMax=[]  SumI1OutMin=[]  SumI1OutMax=[]  SumI2OutMin=[]  SumI2OutMax=[]  SumI3OutMin=[]  SumI3OutMax=[]  SumDOutMin=[]  SumDOutMax=[]  SaturationOutMin=[]  SaturationOutMax=[]  IntegratorContinuousStateAttributes=''  IntegratorStateMustResolveToSignalObject=off  IntegratorRTWStateStorageClass=Auto  FilterContinuousStateAttributes=''  FilterStateMustResolveToSignalObject=off  FilterRTWStateStorageClass=Auto  DifferentiatorICPrevScaledInput=0  DifferentiatorOutMin=[]  DifferentiatorOutMax=[]  FilterDiffOutCoefMin=[]  FilterDiffOutCoefMax=[]  SumDenOutMin=[]  SumDenOutMax=[]  SumNumOutMin=[]  SumNumOutMax=[]  ReciprocalOutMin=[]  ReciprocalOutMax=[]  DivideOutMin=[]  DivideOutMax=[]  TunerSelectOption=Transfer Function Based (PID Tuner App)
  cyemi_{669..676} (8 alike) : DataTypeConversion  OutDataTypeStr=double
  cfblk2 : Outport
  cfblk12 : Outport  Port=2
  wires:
  cfblk1/1 -> cfblk12/1
  cfblk9/1 -> cfblk2/1
  cyemi_669/1 -> cfblk10/1
  cfblk5/1 -> cyemi_669/1
  cyemi_670/1 -> cfblk3/1
  cfblk10/1 -> cyemi_670/1
  cyemi_671/1 -> cfblk4/1
  cfblk8/1 -> cyemi_671/1
  cyemi_672/1 -> cfblk5/1
  cfblk6/1 -> cyemi_672/1
  cyemi_673/1 -> cfblk6/1
  cfblk4/1 -> cyemi_673/1
  cyemi_674/1 -> cfblk7/1
  cfblk3/1 -> cyemi_674/1
  cyemi_675/1 -> cfblk8/1
  cfblk11/1 -> cyemi_675/1
  cyemi_676/1 -> cfblk9/1
  cfblk7/1 -> cyemi_676/1

== system sampleModel7424_pp_1_1/cfblk145/cfblk20 ==
  cfblk1 : Inport
  cfblk10 : Inport  Port=2
  cfblk11 : Inport  Port=3
  cfblk12 : Inport  Port=4
  cfblk13 : Inport  Port=5
  Action Port : ActionPort  ActionType=else
  cfblk3 : simulink/Discrete/Difference  ICPrevInput=0.0  OutMin=[]  OutMax=[]  OutDataTypeStr=double  OutputDataTypeScalingMode=double  OutDataType=fixdt(1, 16)  OutScaling=2^-10  DoSatur=off
  cfblk4 : DiscreteFir
  cfblk5 : Delay
  cfblk6 : Delay
  cfblk7 : Delay  DelayLengthSource=Input port
      settings: InputPortMap=u0,p1
  cfblk8 : Delay  ShowEnablePort=on
      settings: InputPortMap=u0,e6
  cfblk9 : simulink/Discrete/Transfer Fcn Lead or Lag  PoleZ=0.95  ZeroZ=0.75  ICPrevOutput=0.0  ICPrevInput=0.0  DoSatur=off
      settings: SourceProductName=Simulink  SourceProductBaseCode=SL
  cyemi_{682..690} (9 alike) : DataTypeConversion  OutDataTypeStr=double
  cfblk2 : Outport
  cfblk14 : Outport  Port=2
  cfblk15 : Outport  Port=3
  wires:
  cfblk1/1 -> cfblk15/1
  cfblk12/1 -> cfblk2/1
  cfblk3/1 -> cfblk14/1
  cyemi_682/1 -> cfblk3/1
  cfblk5/1 -> cyemi_682/1
  cyemi_683/1 -> cfblk4/1
  cfblk6/1 -> cyemi_683/1
  cyemi_684/1 -> cfblk5/1
  cfblk9/1 -> cyemi_684/1
  cyemi_685/1 -> cfblk6/1
  cfblk11/1 -> cyemi_685/1
  cyemi_686/1 -> cfblk7/1
  cfblk4/1 -> cyemi_686/1
  cyemi_687/1 -> cfblk7/2
  cfblk10/1 -> cyemi_687/1
  cyemi_688/1 -> cfblk8/1
  cfblk13/1 -> cyemi_688/1
  cyemi_689/1 -> cfblk8/2
  cfblk7/1 -> cyemi_689/1
  cyemi_690/1 -> cfblk9/1
  cfblk8/1 -> cyemi_690/1

== system sampleModel7424_pp_1_1/cfblk148/cfblk18 ==
  cfblk1 : Inport
  Action Port : ActionPort  ActionType=then
  cfblk11 : DataTypeConversion  OutDataTypeStr=double
  cfblk12 : DataTypeConversion  OutDataTypeStr=uint32
  cfblk13 : DataTypeConversion  OutDataTypeStr=uint32
  cfblk14 : DataTypeConversion  OutDataTypeStr=double
  cfblk3 : DiscreteFir
  cfblk4 : simulink/Continuous/PID Controller  Controller=PID  TimeDomain=Discrete-time  SampleTime=-1  IntegratorMethod=Forward Euler  FilterMethod=Forward Euler  Form=Parallel  UseFilter=on  ControllerParametersSource=internal  P=1  I=1  D=0  N=100  InitialConditionSource=internal  InitialConditionForIntegrator=0  InitialConditionForFilter=0  ExternalReset=none  LimitOutput=off  UpperSaturationLimit=inf  LowerSaturationLimit=-inf  LinearizeAsGain=off  AntiWindupMode=none  Kb=1  TrackingMode=off  Kt=1  PParamMin=[]  PParamMax=[]  IParamMin=[]  IParamMax=[]  DParamMin=[]  DParamMax=[]  NParamMin=[]  NParamMax=[]  KbParamMin=[]  KbParamMax=[]  KtParamMin=[]  KtParamMax=[]  POutMin=[]  POutMax=[]  IOutMin=[]  IOutMax=[]  DOutMin=[]  DOutMax=[]  NOutMin=[]  NOutMax=[]  KbOutMin=[]  KbOutMax=[]  KtOutMin=[]  KtOutMax=[]  IntegratorOutMin=[]  IntegratorOutMax=[]  FilterOutMin=[]  FilterOutMax=[]  SumOutMin=[]  SumOutMax=[]  SumI1OutMin=[]  SumI1OutMax=[]  SumI2OutMin=[]  SumI2OutMax=[]  SumI3OutMin=[]  SumI3OutMax=[]  SumDOutMin=[]  SumDOutMax=[]  SaturationOutMin=[]  SaturationOutMax=[]  IntegratorContinuousStateAttributes=''  IntegratorStateMustResolveToSignalObject=off  IntegratorRTWStateStorageClass=Auto  FilterContinuousStateAttributes=''  FilterStateMustResolveToSignalObject=off  FilterRTWStateStorageClass=Auto  DifferentiatorICPrevScaledInput=0  DifferentiatorOutMin=[]  DifferentiatorOutMax=[]  FilterDiffOutCoefMin=[]  FilterDiffOutCoefMax=[]  SumDenOutMin=[]  SumDenOutMax=[]  SumNumOutMin=[]  SumNumOutMax=[]  ReciprocalOutMin=[]  ReciprocalOutMax=[]  DivideOutMin=[]  DivideOutMax=[]  TunerSelectOption=Transfer Function Based (PID Tuner App)
  cfblk5 : DiscreteZeroPole  Poles=[0 0.5]  Gain=1  SampleTime=-1
  cfblk6 : DiscreteFir
  cfblk7 : DiscreteTransferFcn
  cfblk8 : DiscreteStateSpace  SampleTime=-1
  cyemi_743 : DataTypeConversion  OutDataTypeStr=uint32
  cyemi_{744..752} (9 alike) : DataTypeConversion  OutDataTypeStr=double
  cfblk2 : Outport
  cfblk9 : Outport  Port=2
  cfblk10 : Outport  Port=3
  wires:
  cfblk3/1 -> cyemi_746/1, cyemi_752/1
  cfblk5/1 -> cfblk9/1, cyemi_751/1
  cfblk12/1 -> cfblk2/1
  cfblk13/1 -> cfblk10/1
  cyemi_743/1 -> cfblk11/1
  cfblk1/1 -> cyemi_743/1
  cyemi_744/1 -> cfblk12/1
  cfblk8/1 -> cyemi_744/1
  cyemi_745/1 -> cfblk13/1
  cfblk4/1 -> cyemi_745/1
  cyemi_746/1 -> cfblk14/1
  cyemi_747/1 -> cfblk3/1
  cfblk6/1 -> cyemi_747/1
  cyemi_748/1 -> cfblk4/1
  cfblk14/1 -> cyemi_748/1
  cyemi_749/1 -> cfblk5/1
  cfblk11/1 -> cyemi_749/1
  cyemi_750/1 -> cfblk6/1
  cfblk7/1 -> cyemi_750/1
  cyemi_751/1 -> cfblk7/1
  cyemi_752/1 -> cfblk8/1

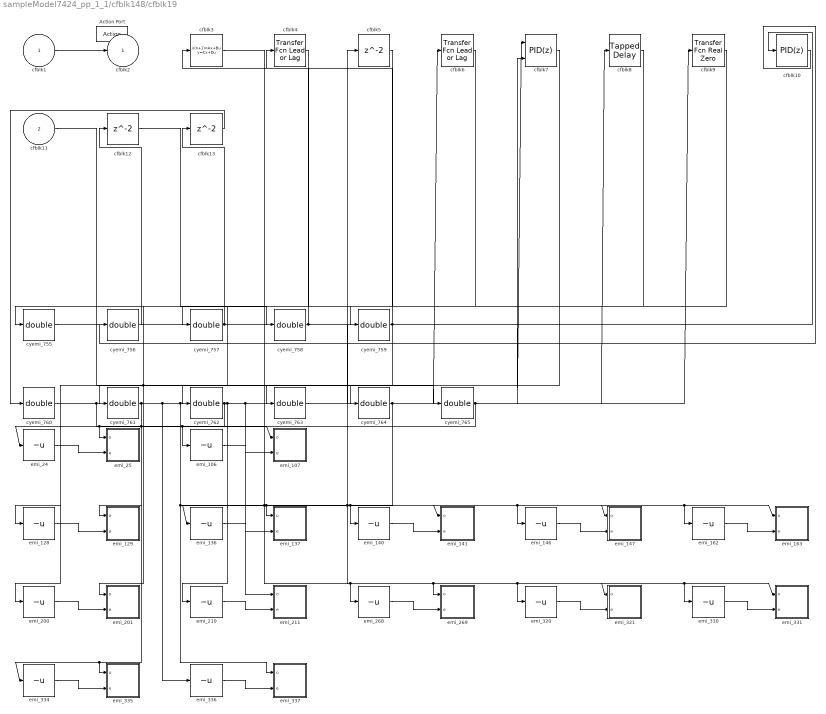
== system sampleModel7424_pp_1_1/cfblk148/cfblk19 ==
  cfblk1 : Inport
  cfblk11 : Inport  Port=2
  Action Port : ActionPort  ActionType=else
  cfblk10 : simulink/Continuous/PID Controller  Controller=PID  TimeDomain=Discrete-time  SampleTime=-1  IntegratorMethod=Forward Euler  FilterMethod=Forward Euler  Form=Parallel  UseFilter=on  ControllerParametersSource=internal  P=1  I=1  D=0  N=100  InitialConditionSource=internal  InitialConditionForIntegrator=0  InitialConditionForFilter=0  ExternalReset=none  LimitOutput=off  UpperSaturationLimit=inf  LowerSaturationLimit=-inf  LinearizeAsGain=off  AntiWindupMode=none  Kb=1  TrackingMode=off  Kt=1  PParamMin=[]  PParamMax=[]  IParamMin=[]  IParamMax=[]  DParamMin=[]  DParamMax=[]  NParamMin=[]  NParamMax=[]  KbParamMin=[]  KbParamMax=[]  KtParamMin=[]  KtParamMax=[]  POutMin=[]  POutMax=[]  IOutMin=[]  IOutMax=[]  DOutMin=[]  DOutMax=[]  NOutMin=[]  NOutMax=[]  KbOutMin=[]  KbOutMax=[]  KtOutMin=[]  KtOutMax=[]  IntegratorOutMin=[]  IntegratorOutMax=[]  FilterOutMin=[]  FilterOutMax=[]  SumOutMin=[]  SumOutMax=[]  SumI1OutMin=[]  SumI1OutMax=[]  SumI2OutMin=[]  SumI2OutMax=[]  SumI3OutMin=[]  SumI3OutMax=[]  SumDOutMin=[]  SumDOutMax=[]  SaturationOutMin=[]  SaturationOutMax=[]  IntegratorContinuousStateAttributes=''  IntegratorStateMustResolveToSignalObject=off  IntegratorRTWStateStorageClass=Auto  FilterContinuousStateAttributes=''  FilterStateMustResolveToSignalObject=off  FilterRTWStateStorageClass=Auto  DifferentiatorICPrevScaledInput=0  DifferentiatorOutMin=[]  DifferentiatorOutMax=[]  FilterDiffOutCoefMin=[]  FilterDiffOutCoefMax=[]  SumDenOutMin=[]  SumDenOutMax=[]  SumNumOutMin=[]  SumNumOutMax=[]  ReciprocalOutMin=[]  ReciprocalOutMax=[]  DivideOutMin=[]  DivideOutMax=[]  TunerSelectOption=Transfer Function Based (PID Tuner App)
  cfblk12 : Delay
  cfblk13 : Delay
  cfblk3 : DiscreteStateSpace  SampleTime=-1
  cfblk4 : simulink/Discrete/Transfer Fcn Lead or Lag  PoleZ=0.95  ZeroZ=0.75  ICPrevOutput=0.0  ICPrevInput=0.0  DoSatur=off
      settings: SourceProductName=Simulink  SourceProductBaseCode=SL
  cfblk5 : Delay
  cfblk6 : simulink/Discrete/Transfer Fcn Lead or Lag  PoleZ=0.95  ZeroZ=0.75  ICPrevOutput=0.0  ICPrevInput=0.0  DoSatur=off
      settings: SourceProductName=Simulink  SourceProductBaseCode=SL
  cfblk7 : simulink/Continuous/PID Controller (2DOF)  Controller=PID  TimeDomain=Discrete-time  SampleTime=-1  IntegratorMethod=Forward Euler  FilterMethod=Forward Euler  Form=Parallel  UseFilter=on  ControllerParametersSource=internal  P=1  I=1  D=0  N=100  b=1  c=1  InitialConditionSource=internal  InitialConditionForIntegrator=0  InitialConditionForFilter=0  ExternalReset=none  LimitOutput=off  UpperSaturationLimit=inf  LowerSaturationLimit=-inf  LinearizeAsGain=off  AntiWindupMode=none  Kb=1  TrackingMode=off  Kt=1  PParamMin=[]  PParamMax=[]  IParamMin=[]  IParamMax=[]  DParamMin=[]  DParamMax=[]  NParamMin=[]  NParamMax=[]  bParamMin=[]  bParamMax=[]  cParamMin=[]  cParamMax=[]  KbParamMin=[]  KbParamMax=[]  KtParamMin=[]  KtParamMax=[]  POutMin=[]  POutMax=[]  IOutMin=[]  IOutMax=[]  DOutMin=[]  DOutMax=[]  NOutMin=[]  NOutMax=[]  bOutMin=[]  bOutMax=[]  cOutMin=[]  cOutMax=[]  KbOutMin=[]  KbOutMax=[]  KtOutMin=[]  KtOutMax=[]  IntegratorOutMin=[]  IntegratorOutMax=[]  FilterOutMin=[]  FilterOutMax=[]  SumOutMin=[]  SumOutMax=[]  Sum1OutMin=[]  Sum1OutMax=[]  Sum2OutMin=[]  Sum2OutMax=[]  Sum3OutMin=[]  Sum3OutMax=[]  SumI1OutMin=[]  SumI1OutMax=[]  SumI2OutMin=[]  SumI2OutMax=[]  SumI3OutMin=[]  SumI3OutMax=[]  SumDOutMin=[]  SumDOutMax=[]  SaturationOutMin=[]  SaturationOutMax=[]  IntegratorContinuousStateAttributes=''  IntegratorStateMustResolveToSignalObject=off  IntegratorRTWStateStorageClass=Auto  FilterContinuousStateAttributes=''  FilterStateMustResolveToSignalObject=off  FilterRTWStateStorageClass=Auto  DifferentiatorICPrevScaledInput=0  DifferentiatorOutMin=[]  DifferentiatorOutMax=[]  FilterDiffOutCoefMin=[]  FilterDiffOutCoefMax=[]  SumDenOutMin=[]  SumDenOutMax=[]  SumNumOutMin=[]  SumNumOutMax=[]  ReciprocalOutMin=[]  ReciprocalOutMax=[]  DivideOutMin=[]  DivideOutMax=[]  TunerSelectOption=Transfer Function Based (PID Tuner App)
  cfblk8 : simulink/Discrete/Tapped Delay  vinit=0.0  samptime=-1  NumDelays=1  DelayOrder=Oldest  includeCurrent=off
  cfblk9 : simulink/Discrete/Transfer Fcn Real Zero  ZeroZ=0.75  ICPrevInput=0.0  DoSatur=off
      settings: SourceProductName=Simulink  SourceProductBaseCode=SL
  cyemi_{755..765} (11 alike) : DataTypeConversion  OutDataTypeStr=double
  emi_{24,106,128,136,140,146,162,200,210,268,320,330,334,336} (14 alike) : UnaryMinus
  emi_107 : MATLAB Function  TreatAsAtomicUnit=on
  emi_129 : MATLAB Function  TreatAsAtomicUnit=on
  emi_137 : MATLAB Function  TreatAsAtomicUnit=on
  emi_141 : MATLAB Function  TreatAsAtomicUnit=on
  emi_147 : MATLAB Function  TreatAsAtomicUnit=on
  emi_163 : MATLAB Function  TreatAsAtomicUnit=on
  emi_201 : MATLAB Function  TreatAsAtomicUnit=on
  emi_211 : MATLAB Function  TreatAsAtomicUnit=on
  emi_25 : MATLAB Function  TreatAsAtomicUnit=on
  emi_269 : MATLAB Function  TreatAsAtomicUnit=on
  emi_321 : MATLAB Function  TreatAsAtomicUnit=on
  emi_331 : MATLAB Function  TreatAsAtomicUnit=on
  emi_335 : MATLAB Function  TreatAsAtomicUnit=on
  emi_337 : MATLAB Function  TreatAsAtomicUnit=on
  cfblk2 : Outport
  wires:
  cfblk1/1 -> cfblk2/1
  cyemi_755/1 -> cfblk10/1
  cfblk6/1 -> cyemi_755/1
  cyemi_756/1 -> cfblk12/1
  cfblk10/1 -> cyemi_756/1
  cyemi_757/1 -> emi_330/1, emi_331/1(o), emi_269/1(o), emi_268/1, emi_140/1, emi_141/1(o), cfblk13/1
  cfblk8/1 -> cyemi_757/1
  cyemi_758/1 -> emi_320/1, emi_321/1(o), emi_162/1, emi_163/1(o), cfblk3/1
  cfblk12/1 -> cyemi_758/1
  cyemi_759/1 -> emi_200/1, emi_201/1(o), cfblk4/1
  cfblk9/1 -> cyemi_759/1
  cyemi_760/1 -> emi_106/1, emi_107/1(o), cfblk5/1
  cfblk13/1 -> cyemi_760/1
  cyemi_761/1 -> emi_334/1, emi_335/1(o), emi_146/1, emi_147/1(o), emi_337/1(o), cfblk6/1, emi_336/1
  cfblk4/1 -> cyemi_761/1
  cyemi_762/1 -> emi_128/1, emi_129/1(o), cfblk7/1, emi_211/1(o), emi_210/1
  cfblk5/1 -> cyemi_762/1
  cyemi_763/1 -> cfblk7/2
  cfblk11/1 -> cyemi_763/1
  cyemi_764/1 -> emi_136/1, emi_137/1(o), cfblk8/1
  cfblk7/1 -> cyemi_764/1
  cyemi_765/1 -> emi_24/1, emi_25/1(o), cfblk9/1
  cfblk3/1 -> cyemi_765/1
  emi_24/1 -> emi_25/2(e)
  emi_106/1 -> emi_107/2(e)
  emi_128/1 -> emi_129/2(e)
  emi_136/1 -> emi_137/2(e)
  emi_140/1 -> emi_141/2(e)
  emi_146/1 -> emi_147/2(e)
  emi_162/1 -> emi_163/2(e)
  emi_200/1 -> emi_201/2(e)
  emi_210/1 -> emi_211/2(e)
  emi_268/1 -> emi_269/2(e)
  emi_320/1 -> emi_321/2(e)
  emi_330/1 -> emi_331/2(e)
  emi_334/1 -> emi_335/2(e)
  emi_336/1 -> emi_337/2(e)

== matlab function sampleModel7424_pp_1_1/cfblk134/emi_3 ==
  data: o input; e input
function  fcn(o, e)
o_inv = o^-1;
e_inv = e^-1;

emsg = 'sampleModel7424_pp_1_1/cfblk134/emi_3';
 
if(o == e)
    assert(o_inv == e_inv, [emsg ' ; o_inv~=e_inv']);
    return;
end
 
if(o_inv > 0)
    assert(e_inv < 0, [emsg ' ; e_inv>=0']);
else
    assert(e_inv > 0, [emsg ' ; e_inv<=0']);
end

== matlab function sampleModel7424_pp_1_1/cfblk142/cfblk17/emi_1 ==
  data: o input; e input
function  fcn(o, e)
o_inv = o^-1;
e_inv = e^-1;

emsg = 'sampleModel7424_pp_1_1/cfblk142/cfblk17/emi_1';
 
if(o == e)
    assert(o_inv == e_inv, [emsg ' ; o_inv~=e_inv']);
    return;
end
 
if(o_inv > 0)
    assert(e_inv < 0, [emsg ' ; e_inv>=0']);
else
    assert(e_inv > 0, [emsg ' ; e_inv<=0']);
end

== matlab function sampleModel7424_pp_1_1/emi_5 ==
  data: o input; e input
function  fcn(o, e)
o_inv = o^-1;
e_inv = e^-1;

emsg = 'sampleModel7424_pp_1_1/emi_5';
 
if(o == e)
    assert(o_inv == e_inv, [emsg ' ; o_inv~=e_inv']);
    return;
end
 
if(o_inv > 0)
    assert(e_inv < 0, [emsg ' ; e_inv>=0']);
else
    assert(e_inv > 0, [emsg ' ; e_inv<=0']);
end

== matlab function sampleModel7424_pp_1_1/cfblk134/emi_7 ==
  data: o input; e input
function  fcn(o, e)
o_inv = o^-1;
e_inv = e^-1;

emsg = 'sampleModel7424_pp_1_1/cfblk134/emi_7';
 
if(o == e)
    assert(o_inv == e_inv, [emsg ' ; o_inv~=e_inv']);
    return;
end
 
if(o_inv > 0)
    assert(e_inv < 0, [emsg ' ; e_inv>=0']);
else
    assert(e_inv > 0, [emsg ' ; e_inv<=0']);
end

== matlab function sampleModel7424_pp_1_1/cfblk142/cfblk19/emi_9 ==
  data: o input; e input
function  fcn(o, e)
o_inv = o^-1;
e_inv = e^-1;

emsg = 'sampleModel7424_pp_1_1/cfblk142/cfblk19/emi_9';
 
if(o == e)
    assert(o_inv == e_inv, [emsg ' ; o_inv~=e_inv']);
    return;
end
 
if(o_inv > 0)
    assert(e_inv < 0, [emsg ' ; e_inv>=0']);
else
    assert(e_inv > 0, [emsg ' ; e_inv<=0']);
end
